simulink model "HIL_Testing_SW_amantest"  (Simulink 7.5)
settings: Solver=ode1  StartTime=0.0  StopTime=Inf  FixedStep=0.001  RelTol=1e-3
PostLoadFcn:
  | , if any(exist('dsrtsu_mdlpostloadfcn', 'file') == [2, 3, 6]), try dsrtsu_mdlpostloadfcn('Execute', bdroot); catch fprintf('Error in PostLoadFcn (dsrtsu_mdlpostloadfcn) for model "%s":\n %s\n', bdroot, lasterr); end, end,
undefined symbols (not defined in the file): CeBSER_Cnt_NumTempAxisPts, ChargeCord, ChargeCord_Control, ChargeToSOCCurr, ChrgCurrLim, CrntSens1Fine, CS_SOCSetPt, CyclerMaxChrgPwr, CyclerMaxDschrgPwr, deltaAhr, Drive_1, Drive_10, Drive_11, Drive_12, Drive_13, Drive_14, Drive_15, Drive_16, Drive_17, Drive_18, Drive_19, Drive_2, Drive_20, Drive_21, Drive_22, Drive_23, Drive_24, Drive_25, Drive_26, Drive_27, Drive_28, Drive_29, Drive_3, Drive_30, Drive_31, Drive_32, Drive_33, Drive_34, Drive_35, Drive_36, Drive_37, Drive_38, Drive_39, Drive_4, Drive_40, Drive_41, Drive_42, Drive_43, Drive_44, Drive_45, Drive_46, Drive_47, Drive_48, Drive_49, Drive_5, Drive_50, Drive_51, Drive_6, Drive_7, Drive_8 ... (+50)
libraries: simulink x129, rtican x50, rti2211sailib x5, rti2211serlib x5, rti2202miolib x3
(part 22 of 23)

== stateflow chart LionsHeart/FeaturePresentation/Down_to_Business/DriveProfile_ModeControl/Pulse/Pulse ==
  state ChrgPulse
    entry:
    Step =1;
    Mode_Cntrl = 2;
    Control_Value=CPower*1000;
    PulseTime = 0;
    du:
    PulseTime = PulseTime + sim_step_time
  state DischrgPulse
    entry:
    Step =1;
    Mode_Cntrl = 2;
    Control_Value=DPower*1000;
    PulseTime = 0;
    du:
    PulseTime = PulseTime + sim_step_time
  state EndTime
    entry:
    Step =2;
    exit:
    Step=0;
  state DirectionDecision
    entry:
    Step =0;
  (default) -> DirectionDecision
  ChrgPulse -> EndTime : [PulseTime >= PulseDuration]
  DischrgPulse -> EndTime : [PulseTime >=PulseDuration]
  DirectionDecision -> ChrgPulse [order 2] : [Direction==1]
  DirectionDecision -> DischrgPulse [order 1] : [Direction==2]
  EndTime -> DirectionDecision : [Step==0]
  data: Control_Value output double; WaitTime output double; Mode_Cntrl output single; Voltage input single; Current input single; sim_step_time input single; ChrgCurrLim input single; DischrgCurrLim input single; Step output single; PulseTime local double; Direction input single; CPower input double; DPower input double; PulseDuration input double

== stateflow chart LionsHeart/FeaturePresentation/Down_to_Business/DriveProfile_ModeControl/Rate/PulseRate ==
  state ChrgPulse
    entry:
    Step =1;
    Mode_Cntrl = 2;
    Control_Value=124*1000;
    PulseTime = 0;
    ChrgCurrLim_Temp = CurrLim;
    du:
    PulseTime = PulseTime + sim_step_time
  state DischrgPulse
    entry:
    Step =1;
    Mode_Cntrl = 2;
    Control_Value=-124*1000;
    PulseTime = 0;
    DischrgCurrLim_Temp = CurrLim;
    du:
    PulseTime = PulseTime + sim_step_time
  state EndTime
    entry:
    Wait=0;
    Mode_Cntrl =3;
    Step =2;
    DischrgCurrLim_Temp = -1*DischrgCurrLim_Cal;
    ChrgCurrLim_Temp = ChrgCurrLim_Cal;
    du:
    Wait=Wait+sim_step_time;
    exit:
    Step=2;
  state DirectionDecision
    entry:
    DischrgCurrLim_Temp = 0;
    ChrgCurrLim_Temp = 0;
    Step =0;
  state WaitForMe
    entry:
    Wait=0;
    Mode_Cntrl =3;
    Step =3;
    du:
    Wait=Wait+sim_step_time;
  state WaitForMe1
    entry:
    Wait=0;
    Mode_Cntrl =2;
    Step =3;
    du:
    Wait=Wait+sim_step_time;
  state WaitForMe2
    entry:
    Wait=0;
    Mode_Cntrl =2;
    Step =3;
    du:
    Wait=Wait+sim_step_time;
  (default) -> DirectionDecision
  ChrgPulse -> WaitForMe : [PulseTime >= PTime]
  DischrgPulse -> WaitForMe : [PulseTime >=PTime]
  DirectionDecision -> WaitForMe1 [order 2] : [Direction==1]
  DirectionDecision -> WaitForMe2 [order 1] : [Direction==2]
  EndTime -> DirectionDecision : [Step==2]
  WaitForMe -> EndTime : [(Wait>=2)]
  WaitForMe2 -> DischrgPulse : [(Wait>=2)]
  WaitForMe1 -> ChrgPulse : [(Wait>=2)]
  data: Control_Value output double; ChrgCurrLim_Temp output double; Mode_Cntrl output single; sim_step_time input single; ChrgCurrLim_Cal input single; DischrgCurrLim_Cal input single; Step output single; PulseTime local double; Direction input single; PTime input double; DischrgCurrLim_Temp output double; CurrLim input double; Wait local double

== stateflow chart LionsHeart/FeaturePresentation/Safety/SafetyCheck ==
  state SafetyCheck
    entry:
    Mode_Cntrl=Mode;
    du:
    Mode_Cntrl=Mode;
    Fault =0;
  state HotTempSafety
    entry:
    Mode_Cntrl= 3;
    Fault =7;
  state ColdTempSafety
    entry:
    Mode_Cntrl= 3;
    Fault = 8;
  state VoltageFloorCell
    entry:
    Mode_Cntrl= 3;
    Fault= 1;
  state VoltageLidCell
    entry:
    Mode_Cntrl= 3;
    Fault = 4;
  state ContactorOpenFault
    entry:
    Mode_Cntrl= 3;
    Fault = 9;
  state Wait_VFC
  state Wait_Hot
  state Wait_VLC
  state Wait_Cold
  state Wait_Cntctr
  state VoltageFloorPack
    entry:
    Mode_Cntrl= 3;
    Fault= 2;
  state VoltageFloorCycler
    entry:
    Mode_Cntrl= 3;
    Fault= 3;
  state VoltageLidPack
    entry:
    Mode_Cntrl= 3;
    Fault =5;
  state VoltageLidCycler
    entry:
    Mode_Cntrl= 3;
    Fault = 6;
  state Wait_VFP
  state Wait_VFCy
  state Wait_VLP
  state Wait_VLCy
  (default) -> SafetyCheck
  SafetyCheck -> Wait_Hot [order 1] : [(BatTemp>=BatTempHot) && ((ContactorLine==1))]
  HotTempSafety -> SafetyCheck : [Resume==1]
  SafetyCheck -> Wait_Cold [order 5] : [(BatTemp<=BatTempCold) && ((ContactorLine==1))]
  ColdTempSafety -> SafetyCheck : [Resume==1]
  SafetyCheck -> Wait_VFC [order 6] : [(((VoltageMin<=Voltage_Floor_Cell -Safety_FloorOffset)) && (ContactorLine==1) && (SF!=5)&& (MinCell_Enbl==1))]
  VoltageFloorCell -> SafetyCheck : [Resume==1]
  SafetyCheck -> Wait_VLC [order 3] : [(((VoltageMax>=Voltage_Lid_Cell + Safety_LidOffset) & (ContactorLine==1) & (SF!=5) & (MaxCell_Enbl==1)))]
  VoltageLidCell -> SafetyCheck : [Resume==1]
  SafetyCheck -> Wait_Cntctr [order 4] : [ContactorStatus == 1]
  ContactorOpenFault -> SafetyCheck : [Resume==1]
  Wait_VFC -> VoltageFloorCell [order 1] : after(FaultTime,sec)
  Wait_VFC -> SafetyCheck [order 2] : [(VoltageMin>Voltage_Floor_Cell-Safety_FloorOffset)]
  Wait_Hot -> HotTempSafety [order 1] : after(FaultTime,sec)
  Wait_VLC -> VoltageLidCell [order 1] : after(FaultTime,sec)
  Wait_Hot -> SafetyCheck [order 2] : [BatTemp<=BatTempHot]
  Wait_VLC -> SafetyCheck [order 2] : [(VoltageMax<=(Voltage_Lid_Cell + Safety_LidOffset))]
  Wait_Cold -> SafetyCheck [order 2] : [BatTemp>=BatTempCold]
  Wait_Cold -> ColdTempSafety [order 1] : after(FaultTime,sec)
  Wait_Cntctr -> ContactorOpenFault [order 1] : after(FaultTime,sec)
  Wait_Cntctr -> SafetyCheck [order 2] : [ContactorStatus ==0]
  SafetyCheck -> Wait_VFP [order 7] : [(((VoltagePack<=Voltage_Floor -Safety_FloorOffset)) && (ContactorLine==1) && (SF!=5)&& (PackSensor==1))]
  Wait_VFP -> VoltageFloorPack [order 1] : after(FaultTime,sec)
  VoltageFloorPack -> SafetyCheck : [Resume==1]
  Wait_VFP -> SafetyCheck [order 2] : [(VoltagePack>Voltage_Floor-Safety_FloorOffset)]
  SafetyCheck -> Wait_VFCy [order 8] : [(((VoltageCycler<=Voltage_Floor -Safety_FloorOffset)) && (ContactorLine==1) && (SF!=5))]
  Wait_VFCy -> VoltageFloorCycler [order 1] : after(FaultTime,sec)
  Wait_VFCy -> SafetyCheck [order 2] : [(VoltageCycler>Voltage_Floor-Safety_FloorOffset)]
  VoltageFloorCycler -> SafetyCheck : [Resume==1]
  Wait_VLP -> VoltageLidPack [order 1] : after(FaultTime,sec)
  VoltageLidPack -> SafetyCheck : [Resume==1]
  SafetyCheck -> Wait_VLP [order 2] : [(((VoltagePack>=Voltage_Lid + Safety_LidOffset) & (ContactorLine==1) & (SF!=5) & (PackSensor==1)))]
  Wait_VLP -> SafetyCheck [order 2] : [(VoltagePack<=(Voltage_Lid+Safety_LidOffset))]
  Wait_VLCy -> VoltageLidCycler [order 1] : after(FaultTime,sec)
  VoltageLidCycler -> SafetyCheck : [Resume==1]
  SafetyCheck -> Wait_VLCy [order 9] : [(((VoltageCycler>=Voltage_Lid + Safety_LidOffset) & (ContactorLine==1) & (SF!=5)))]
  Wait_VLCy -> SafetyCheck [order 2] : [(VoltageCycler<=(Voltage_Lid+Safety_LidOffset))]
  data: BatTemp input single; VoltageMin input double; VoltageMax input double; Mode_Cntrl output double; BatTempHot input single; BatTempCold input single; Voltage_Floor input single; Voltage_Lid input single; Mode input single; Fault output double; Resume input double; ContactorLine input boolean; ContactorStatus input boolean; SF input double; Voltage_Floor_Cell input double; VoltagePack input double; Voltage_Lid_Cell input double; FaultTime input double; Safety_FloorOffset input double; Safety_LidOffset input double; VoltageCycler input double; MaxCell_Enbl input double; MinCell_Enbl input double; PackSensor input double
